simulink model "ContinuousTxModel"  (R2026a)
settings: Solver=FixedStepDiscrete  StopTime=1000
libraries: hdlsllib x7, simulink x1, dsphdlsigops2 x1
settings Model: DataTypeOverride=Off  Creator=jiemingx  LastModifiedBy=jiemingx
settings OptimizationCC: ConditionallyExecuteInputs=off  InheritOutputTypeSmallerThanSingle=on
settings DebuggingCC: ArtificialAlgebraicLoopMsg=error  MergeDetectMultiDrivingBlocksExec=error  SingleTaskRateTransMsg=error
settings HardwareCC: ProdHWDeviceType=ASIC/FPGA->ASIC/FPGA  TargetBitPerLong=64.0  TargetBitPerPointer=64.0  TargetBitPerSizeT=64.0  TargetBitPerPtrDiffT=64.0  TargetLongLongMode=on  TargetIntDivRoundTo=Zero  TargetEndianess=LittleEndian  TargetWordSize=64.0  TargetHWDeviceType=Custom Processor->MATLAB Host Computer  ProdEqTarget=off
settings ModelReferenceCC: PropagateSignalLabelsOutOfModel=on

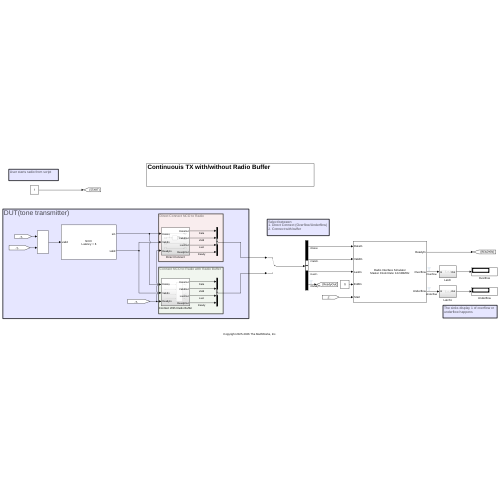
[thumbnail: Simulink's stored preview of the top-level diagram]
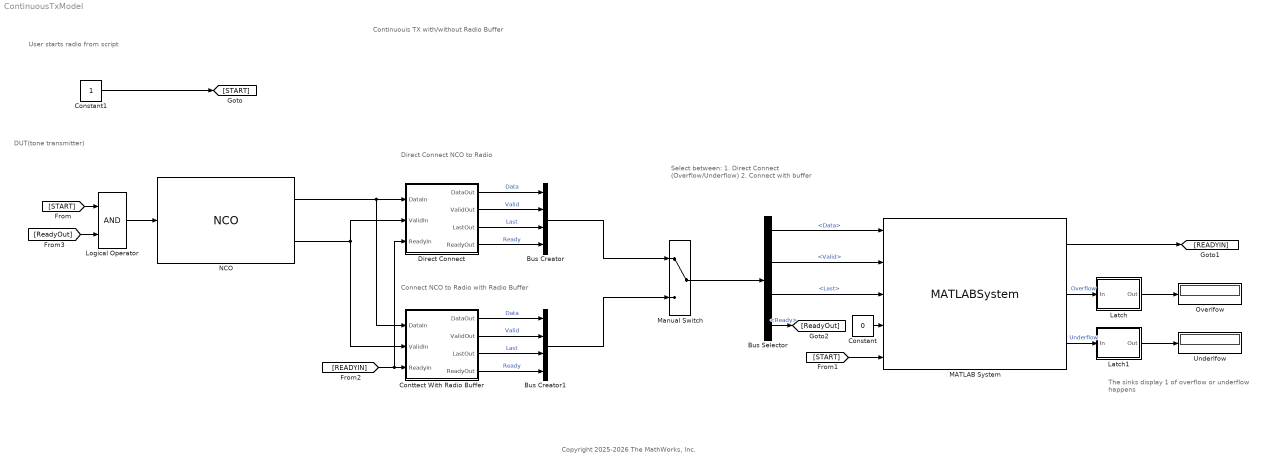
== system ContinuousTxModel ==
  note: User starts radio from script
  note: The sinks display 1 of overflow or
      | underflow happens
  note: Select between:
      | 1. Direct Connect (Overflow/Underflow)
      | 2. Connect with buffer
  note: DUT(tone transmitter)
  note: Continuouis TX with/without Radio Buffer
  note: Direct Connect NCO to Radio
  note: Connect NCO to Radio with Radio Buffer
  note: Copyright 2025-2026 The MathWorks, Inc.
  Bus Creator : BusCreator  Inputs=4
  Bus Creator1 : BusCreator  Inputs=4
  Bus Selector : BusSelector  OutputSignals=Data,Valid,Last,Ready
  Constant : Constant  Value=0  OutDataTypeStr=boolean  SampleTime=1
  Constant1 : Constant  OutDataTypeStr=boolean  SampleTime=1
  Conttect With Radio Buffer : Subsystem
  Direct Connect : Subsystem
  Latch : Subsystem
  Latch1 : Subsystem
  Logical Operator : Logic  AllPortsSameDT=off  OutDataTypeStr=boolean
  MATLAB System : MATLABSystem  System=RadioInterfaceSim  Device=N310  TXRX=TX  ClockSource=Radio  SampleRate=61.44e6  DUTClockRate=61.44e6  InputDataSource=[ 1, 2, 3 ]  SimulateUsing=Interpreted execution  ClockUncertainty=off  Uncertainty=0  Jitter=0
      mask Type: RadioInterfaceSim
  Manual Switch : ManualSwitch
  NCO : dsphdlsigops2/NCO  PhaseIncrementSource=Property  PhaseIncrement=100  Frequency=510  FreqResolution=0.05  SamplingFreq=4000  PhaseOffsetSource=Property  PhaseOffset=0  PhaseOffsetR=pi / 3  DitherSource=Property  NumDitherBits=4  SamplesPerFrame=1  LUTCompress=off  ResetAction=off  Waveform=Sine  PhasePort=off  SimulateUsing=Code generation  AccumulatorWL=16  PhaseQuantization=on  NumQuantizerAccumulatorBits=12  OutputDataType=Binary point scaling  OutputWL=16  OutputFL=14
  Overlfow : Display
  Underlfow : Display
  wires:
  NCO/2 -> Conttect With Radio Buffer/2(ValidIn), Direct Connect/2(ValidIn)
  NCO/1 -> Conttect With Radio Buffer/1(DataIn), Direct Connect/1(DataIn)
  Constant/1 -> MATLAB System/4
  Constant1/1 -> [START]
  Logical Operator/1 -> NCO/1
  [START] -> Logical Operator/1
  [START] -> MATLAB System/5
  Direct Connect/4(ReadyOut) -> Bus Creator/4  "Ready"
  Conttect With Radio Buffer/4(ReadyOut) -> Bus Creator1/4  "Ready"
  Conttect With Radio Buffer/1(DataOut) -> Bus Creator1/1  "Data"
  Conttect With Radio Buffer/2(ValidOut) -> Bus Creator1/2  "Valid"
  Conttect With Radio Buffer/3(LastOut) -> Bus Creator1/3  "Last"
  MATLAB System/1 -> [READYIN]
  [READYIN] -> Direct Connect/3(ReadyIn), Conttect With Radio Buffer/3(ReadyIn)
  Bus Creator/1 -> Manual Switch/1
  Bus Creator1/1 -> Manual Switch/2
  Bus Selector/1 -> MATLAB System/1  "<Data>"
  Bus Selector/2 -> MATLAB System/2  "<Valid>"
  Bus Selector/3 -> MATLAB System/3  "<Last>"
  Manual Switch/1 -> Bus Selector/1
  Bus Selector/4 -> [ReadyOut]  "<Ready>"
  [ReadyOut] -> Logical Operator/2
  MATLAB System/2 -> Latch/1(In)  "Overflow"
  MATLAB System/3 -> Latch1/1(In)  "Underflow"
  Latch/1(Out) -> Overlfow/1
  Latch1/1(Out) -> Underlfow/1
  Direct Connect/3(LastOut) -> Bus Creator/3  "Last"
  Direct Connect/2(ValidOut) -> Bus Creator/2  "Valid"
  Direct Connect/1(DataOut) -> Bus Creator/1  "Data"

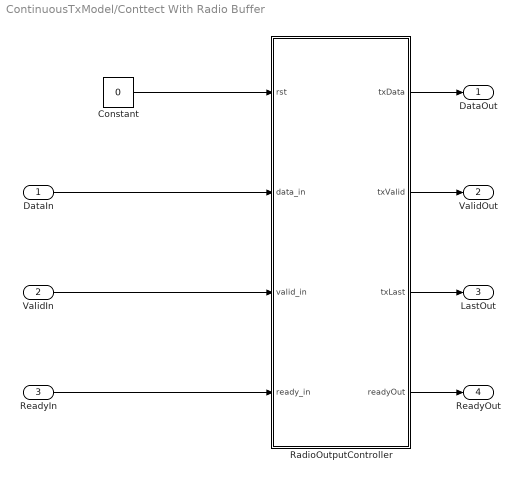
== system ContinuousTxModel/Conttect With Radio Buffer ==
  DataIn : Inport
  ValidIn : Inport  Port=2
  ReadyIn : Inport  Port=3
  Constant : Constant  Value=0  OutDataTypeStr=boolean  SampleTime=-1
  RadioOutputController : Subsystem
  DataOut : Outport
  ValidOut : Outport  Port=2
  LastOut : Outport  Port=3
  ReadyOut : Outport  Port=4
  wires:
  DataIn/1 -> RadioOutputController/2(data_in)
  ValidIn/1 -> RadioOutputController/3(valid_in)
  ReadyIn/1 -> RadioOutputController/4(ready_in)
  RadioOutputController/2(txValid) -> ValidOut/1
  RadioOutputController/1(txData) -> DataOut/1
  RadioOutputController/3(txLast) -> LastOut/1
  Constant/1 -> RadioOutputController/1(rst)
  RadioOutputController/4(readyOut) -> ReadyOut/1

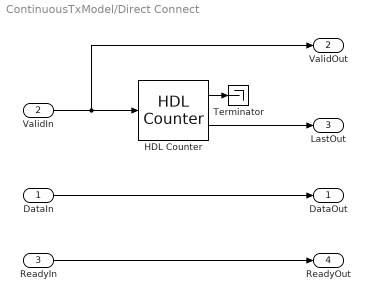
== system ContinuousTxModel/Direct Connect ==
  DataIn : Inport
  ValidIn : Inport  Port=2
  ReadyIn : Inport  Port=3
  HDL Counter : hdlsllib/Sources/HDL Counter  CountType=Free running  CountInit=0  CountStep=1  CountMax=25  CountFromType=Initial value  CountFrom=0  CountResetPort=off  CountLoadPort=off  CountEnbPort=on  CountDirPort=off  CountHitOutputPort=on  CountDataType=Unsigned  CountWordLen=8  CountFracLen=0  CountSampTime=1
  Terminator : Terminator
  DataOut : Outport
  ValidOut : Outport  Port=2
  LastOut : Outport  Port=3
  ReadyOut : Outport  Port=4
  wires:
  HDL Counter/1 -> Terminator/1
  HDL Counter/2 -> LastOut/1
  DataIn/1 -> DataOut/1
  ValidIn/1 -> ValidOut/1, HDL Counter/1
  ReadyIn/1 -> ReadyOut/1

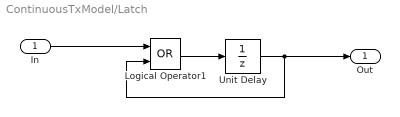
== system ContinuousTxModel/Latch ==
  In : Inport
  Logical Operator1 : Logic  Operator=OR  AllPortsSameDT=off  OutDataTypeStr=boolean
  Unit Delay : UnitDelay  SampleTime=-1
  Out : Outport
  wires:
  Unit Delay/1 -> Out/1, Logical Operator1/2
  In/1 -> Logical Operator1/1
  Logical Operator1/1 -> Unit Delay/1

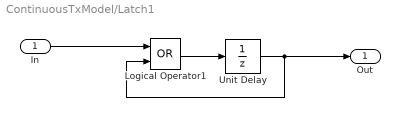
== system ContinuousTxModel/Latch1 ==
  In : Inport
  Logical Operator1 : Logic  Operator=OR  AllPortsSameDT=off  OutDataTypeStr=boolean
  Unit Delay : UnitDelay  SampleTime=-1
  Out : Outport
  wires:
  Unit Delay/1 -> Out/1, Logical Operator1/2
  In/1 -> Logical Operator1/1
  Logical Operator1/1 -> Unit Delay/1

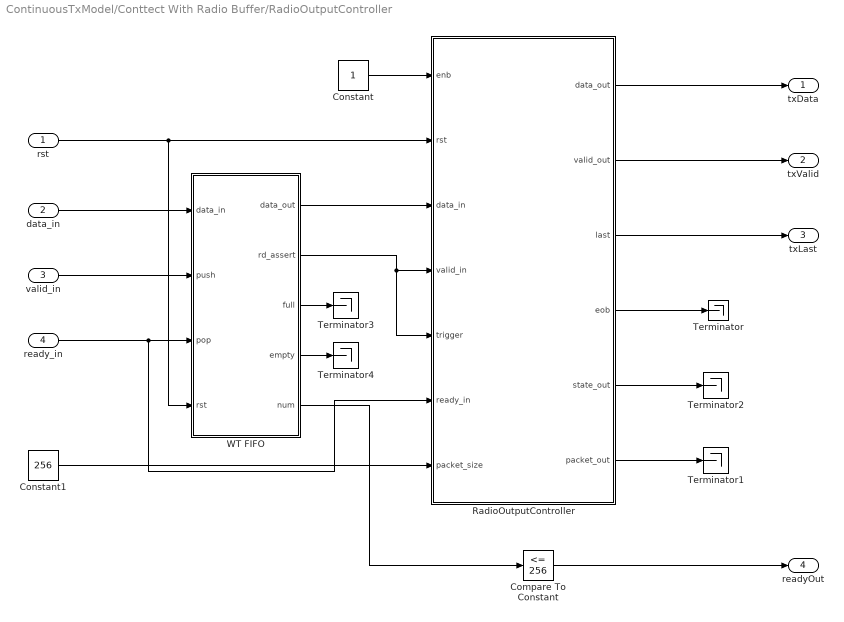
== system ContinuousTxModel/Conttect With Radio Buffer/RadioOutputController ==
  rst : Inport
  data_in : Inport  Port=2
  valid_in : Inport  Port=3
  ready_in : Inport  Port=4
  Compare To Constant : simulink/Logic and Bit Operations/Compare To Constant  relop=<=  const=256  OutDataTypeStr=boolean
  Constant : Constant  OutDataTypeStr=boolean  SampleTime=-1
  Constant1 : Constant  Value=256  OutDataTypeStr=uint16  SampleTime=-1
  RadioOutputController : MATLAB Function  TreatAsAtomicUnit=on  mask{SKID_BUFF_SIZE=8}
      mask prompts: SKID_BUFF_SIZE "Skid Buffer Size"
  Terminator{,1..4} (5 alike) : Terminator
  WT FIFO : Subsystem  mask{depth=10}
      mask prompts: depth "FIFO Depth"
  txData : Outport
  txValid : Outport  Port=2
  txLast : Outport  Port=3
  readyOut : Outport  Port=4
  wires:
  RadioOutputController/4(eob) -> Terminator/1
  WT FIFO/4(empty) -> Terminator4/1
  Constant/1 -> RadioOutputController/1(enb)
  data_in/1 -> WT FIFO/1(data_in)
  rst/1 -> WT FIFO/4(rst), RadioOutputController/2(rst)
  WT FIFO/1(data_out) -> RadioOutputController/3(data_in)
  RadioOutputController/6(packet_out) -> Terminator1/1
  ready_in/1 -> RadioOutputController/6(ready_in), WT FIFO/3(pop)
  RadioOutputController/5(state_out) -> Terminator2/1
  Constant1/1 -> RadioOutputController/7(packet_size)
  WT FIFO/2(rd_assert) -> RadioOutputController/5(trigger), RadioOutputController/4(valid_in)
  RadioOutputController/1(data_out) -> txData/1
  WT FIFO/3(full) -> Terminator3/1
  valid_in/1 -> WT FIFO/2(push)
  WT FIFO/5(num) -> Compare To Constant/1
  RadioOutputController/2(valid_out) -> txValid/1
  RadioOutputController/3(last) -> txLast/1
  Compare To Constant/1 -> readyOut/1

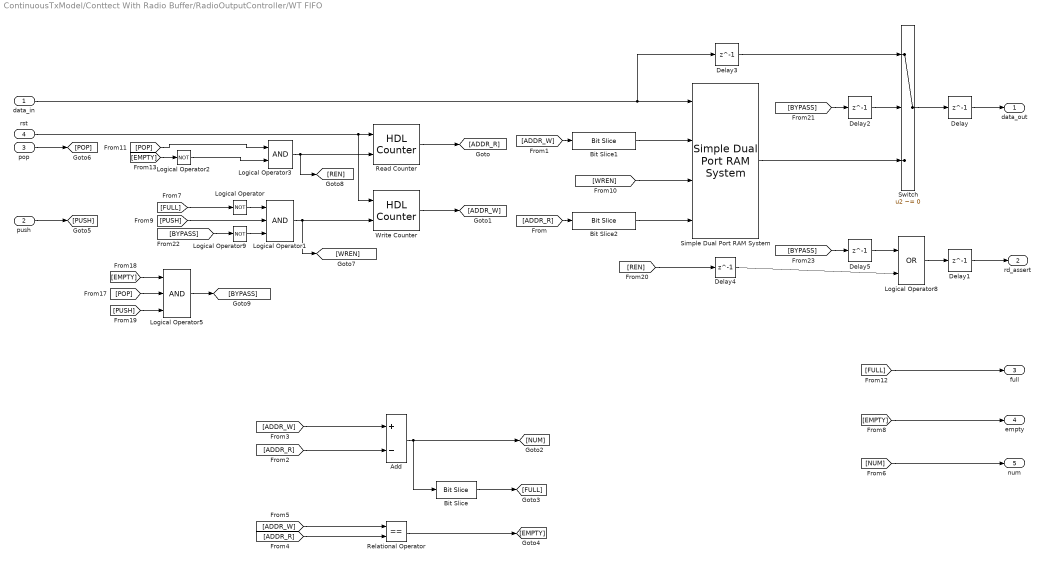
== system ContinuousTxModel/Conttect With Radio Buffer/RadioOutputController/WT FIFO ==
  data_in : Inport
  push : Inport  Port=2
  pop : Inport  Port=3
  rst : Inport  Port=4
  Add : Sum  Inputs=+-  OutDataTypeStr=Inherit: Same as accumulator
  Bit Slice : hdlsllib/Logic and Bit Operations/Bit Slice  lidx=depth  ridx=depth
  Bit Slice1 : hdlsllib/Logic and Bit Operations/Bit Slice  lidx=depth-1  ridx=0
  Bit Slice2 : hdlsllib/Logic and Bit Operations/Bit Slice  lidx=depth-1  ridx=0
  Delay{,1..5} (6 alike) : Delay  DelayLength=1
  Logical Operator : Logic  Operator=NOT  IconShape=distinctive  AllPortsSameDT=off  OutDataTypeStr=boolean
  Logical Operator1 : Logic  Inputs=3  IconShape=distinctive  AllPortsSameDT=off  OutDataTypeStr=boolean
  Logical Operator2 : Logic  Operator=NOT  IconShape=distinctive  AllPortsSameDT=off  OutDataTypeStr=boolean
  Logical Operator3 : Logic  IconShape=distinctive  AllPortsSameDT=off  OutDataTypeStr=boolean
  Logical Operator5 : Logic  Inputs=3  IconShape=distinctive  AllPortsSameDT=off  OutDataTypeStr=boolean
  Logical Operator8 : Logic  Operator=OR  IconShape=distinctive  AllPortsSameDT=off  OutDataTypeStr=boolean
  Logical Operator9 : Logic  Operator=NOT  IconShape=distinctive  AllPortsSameDT=off  OutDataTypeStr=boolean
  Read Counter : hdlsllib/Sources/HDL Counter  CountType=Free running  CountInit=0  CountStep=1  CountMax=25  CountFromType=Initial value  CountFrom=0  CountResetPort=on  CountLoadPort=off  CountEnbPort=on  CountDirPort=off  CountHitOutputPort=off  CountDataType=Unsigned  CountWordLen=depth+1  CountFracLen=0  CountSampTime=1
  Relational Operator : RelationalOperator  Operator===  OutDataTypeStr=boolean  RndMeth=Simplest  InputSameDT=off
  Simple Dual Port RAM System : hdlsllib/HDL RAMs/Simple Dual Port RAM System  RAMType=Simple dual port  AsyncRead=off  WriteOutputValue=New data  RAMInitialValue=0  allowBusInputs=off  WritesHaveOutput=on  NumReads=0  NumWrites=1  SimulateUsing=Code generation  ModelRAMDelay=on  VectorAccess=Parallel
  Switch : Switch  Criteria=u2 ~= 0  SaturateOnIntegerOverflow=off  InputSameDT=off
  Write Counter : hdlsllib/Sources/HDL Counter  CountType=Free running  CountInit=0  CountStep=1  CountMax=25  CountFromType=Initial value  CountFrom=0  CountResetPort=on  CountLoadPort=off  CountEnbPort=on  CountDirPort=off  CountHitOutputPort=off  CountDataType=Unsigned  CountWordLen=depth+1  CountFracLen=0  CountSampTime=1
  data_out : Outport
  rd_assert : Outport  Port=2
  full : Outport  Port=3
  empty : Outport  Port=4
  num : Outport  Port=5
  wires:
  Delay5/1 -> Logical Operator8/1
  Delay4/1 -> Logical Operator8/2
  [BYPASS] -> Delay5/1
  [REN] -> Delay4/1
  [BYPASS] -> Logical Operator9/1
  Logical Operator5/1 -> [BYPASS]
  Delay3/1 -> Switch/1
  Logical Operator9/1 -> Logical Operator1/3
  Delay2/1 -> Switch/2
  Simple Dual Port RAM System/1 -> Switch/3
  Delay1/1 -> rd_assert/1
  Logical Operator8/1 -> Delay1/1
  [EMPTY] -> Logical Operator5/1
  [POP] -> Logical Operator5/2
  [PUSH] -> Logical Operator5/3
  Delay/1 -> data_out/1
  Switch/1 -> Delay/1
  [BYPASS] -> Delay2/1
  [WREN] -> Simple Dual Port RAM System/3
  [ADDR_W] -> Relational Operator/1
  [ADDR_R] -> Relational Operator/2
  Add/1 -> Bit Slice/1, [NUM]
  Logical Operator2/1 -> Logical Operator3/2
  [EMPTY] -> Logical Operator2/1
  [POP] -> Logical Operator3/1
  Logical Operator3/1 -> [REN], Read Counter/2
  Bit Slice2/1 -> Simple Dual Port RAM System/4
  Bit Slice1/1 -> Simple Dual Port RAM System/2
  [ADDR_R] -> Bit Slice2/1
  [NUM] -> num/1
  Relational Operator/1 -> [EMPTY]
  Write Counter/1 -> [ADDR_W]
  [ADDR_W] -> Bit Slice1/1
  [FULL] -> Logical Operator/1
  data_in/1 -> Simple Dual Port RAM System/1, Delay3/1
  Bit Slice/1 -> [FULL]
  Read Counter/1 -> [ADDR_R]
  [FULL] -> full/1
  [ADDR_R] -> Add/2
  rst/1 -> Read Counter/1, Write Counter/1
  [PUSH] -> Logical Operator1/2
  Logical Operator/1 -> Logical Operator1/1
  [ADDR_W] -> Add/1
  Logical Operator1/1 -> [WREN], Write Counter/2
  [EMPTY] -> empty/1
  push/1 -> [PUSH]
  pop/1 -> [POP]

== matlab function ContinuousTxModel/Conttect With Radio Buffer/RadioOutputController/RadioOutputController ==
  data: data_out output; valid_out output; last output; eob output; enb input; rst input boolean; data_in input; valid_in input; trigger input; ready_in input; state_out output; packet_size input; packet_out output; SKID_BUFF_SIZE parameter
function [data_out, valid_out, last, eob, state_out, packet_out] = RadioOutput_Ctrl(enb, rst, data_in, valid_in, trigger, ready_in, packet_size, SKID_BUFF_SIZE)
%#codegen
%% @param out
% data_out:    data output
% valid_out:   Valid output data from DUT
% last:        Last signal of each packet
% eob:         end of burst indicator
% state_out:   Data packager state
% packet_out:  Current number of samples per packet
%% @param in
% enb:         Data pack enable
% rst:         Reset system to IDLE
% data_in:     Data input
% valid_in:    Valid input
% packet_size  Required number of samples per packet

% +---------------+-------------------------------------------+
% | IDLE          | REC            | FINISH                   |
% +---------------+-------------------------------------------+
% | System idle,  | Record a fixed | Current recording        |
% | initial state | number of data | finishes, wait for reset |
% +---------------+-------------------------------------------+
IDLE = ufi(0,3,0);
REC = ufi(1,3,0);
FINISH = ufi(4,3,0);

persistent state;  % system state register
persistent counter_reg;  % number of recorded samples counter
persistent packet_size_reg;
persistent counter_last_reg;  % number of samples of current recorded packet counter
persistent buff;
persistent r;
persistent w;
BUFF_COUNTER_DEPTH = ceil(log2(SKID_BUFF_SIZE))+1;

if(isempty(state))
    counter_reg = ufi(0,32,0);
    packet_size_reg = ufi(256,16,0);
    counter_last_reg = ufi(0,16,0);
    buff = cast(zeros(SKID_BUFF_SIZE,1),'like',data_in);
    state = IDLE;
    r = fi(0,0,BUFF_COUNTER_DEPTH,0,hdlfimath);
    w = fi(0,0,BUFF_COUNTER_DEPTH,0,hdlfimath);
end

state_out = state;
packet_out = packet_size_reg;
rs = bitsliceget(r,BUFF_COUNTER_DEPTH-1,1);
ws = bitsliceget(w,BUFF_COUNTER_DEPTH-1,1);

switch(state)
    case IDLE
        if(valid_in && enb && trigger)
            state_next = REC;
            counter_reg(:) = 1;
            counter_last_reg(:) = 1;
            packet_size_reg(:) = packet_size;
            buff(ws+1) = data_in;
            w(:) = w+1;
        else
            state_next = IDLE;
            w(:) = 0;
            r(:) = 0;
            counter_reg(:) = 0;
            counter_last_reg(:) = 0;
        end
        data_out = buff(rs+1);
        valid_out = false;
        last = false;
        eob = false;

    case REC
        %% Skid buffer
        if(ready_in && valid_in)
            data_out = buff(rs+1);
            r(:) = r + 1;
            buff(ws+1) = data_in;
            w(:) = w+1;
            valid_out_signal = true;
        elseif(~ready_in && valid_in)
            data_out = buff(rs+1);
            buff(ws+1) = data_in;
            w(:) = w + 1;
            valid_out_signal = false;
        elseif(ready_in && ~valid_in)
            if(fi(w-r,0,BUFF_COUNTER_DEPTH,0,hdlfimath)~=1)
                data_out = buff(rs+1);
                r(:) = r + 1;
                valid_out_signal = true;
            else
                data_out = buff(rs+1);
                valid_out_signal = false;
            end
        else
            data_out = buff(rs+1);
            valid_out_signal = false;
        end
        
        if(valid_out_signal)  % current record not finished
            if(counter_last_reg == packet_size_reg)
                counter_last_reg(:) = 1;
                last = true;
            else
                last = false;
                counter_last_reg(:) = counter_last_reg + 1;
            end
            counter_reg(:) = counter_reg + 1;
            eob = false;
            valid_out = true;
            state_next = REC;
        else
            valid_out = false;
            last = false;
            eob = false;
            state_next = REC;
        end

    case FINISH
        state_next = FINISH;
        data_out = buff(rs+1);
        valid_out = false;
        last = false;
        eob = false;
    otherwise
        state_next = IDLE;
        data_out = buff(rs+1);
        valid_out = false;
        last = false;
        eob = false;
end

if(rst)
    state = IDLE;
    counter_reg(:) = 0;
    counter_last_reg(:) = 0;
    buff(:) = 0;
    w(:) = 0;
    r(:) = 0;
else
    state = state_next;
end
